simulink model "biasest_with_control"  (R2023b)
settings: Solver=FixedStepAuto  StartTime=0.0  StopTime=SIMTIME  FixedStep=SIMSTEP  RelTol=1e-3
values from neighbouring files (symbols this model uses):
  A = [z33,    eye(3) ... (first row only)    [bias_est.m]
  Aa = [A, Bv(:,1:3); zeros(3, 9)]    [bias_est.m]
  B = [z33, inv(M)]'    [bias_est.m]
  Ba = [B;zeros(3,3)]    [bias_est.m]
  beta_c = deg2rad(1)    [bias_est.m]
  bias = [1e4;1e3;0]    [bias_est.m]
  Bv = [z33 z33 ... (first row only)    [bias_est.m]
  C = [eye(3,6)]    [bias_est.m]
  Ca = [C, zeros(3,3)]    [bias_est.m]
  K2 = Kt2*Q    [bias_est.m]
  L = place(Aa', Ca', lambda_obs)'    [bias_est.m]
  ref = zeros(n_outputs, 1)    [bias_est.m]
  V_curr = 2    [bias_est.m]
  V_wind = 0    [bias_est.m]
  wave_ampl = [0, 0, 0]    [bias_est.m]
  wave_length = [70 70 70]    [bias_est.m]
  x0 = zeros(n_states,1)    [bias_est.m]
  xhat_0 = zeros(n_states+n_aug,1)    [bias_est.m]
undefined symbols (not defined in the file or in its folder): ocean_coeff, wind_coeff
settings Model: Creator=Lorenzo-Desk  LastModifiedBy=Lorenzo-Desk
settings DataIOCC: ReturnWorkspaceOutputs=off

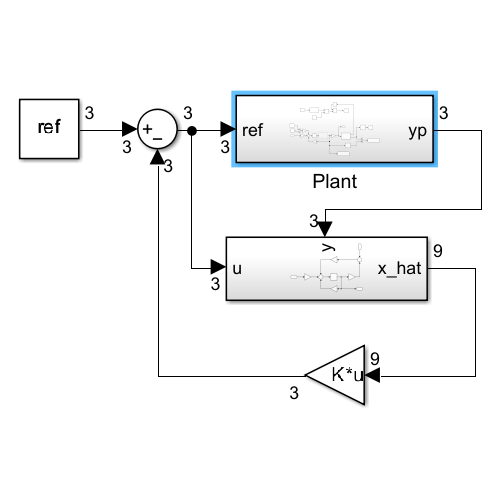
[thumbnail: Simulink's stored preview of the top-level diagram]
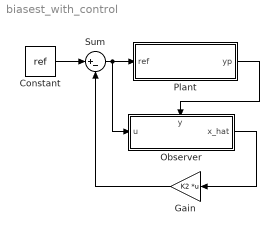
== system biasest_with_control ==
  Constant : Constant  Value=ref
  Gain : Gain  Gain=K2  Multiplication=Matrix(K*u)
  Observer : Subsystem
      settings: PortSchema="{\"entries\":[{\"content\":{\"sides\":[{\"content\":{\"connectorIds\":[\"In1\"]},\"type\":\"ConnectorPlacement.EquallySpacedRectSide\",\"uuid\":\"73eb13a4-821c-44f7-a0c5-8658f41102da\"},{\"content\":{\"connectorIds\":[\"Out1\"],\"side\":\"RIGHT\"},\"type\":\"ConnectorPlacement.EquallySpacedRectSide\",\"uuid\":\"46a10ada-d417-4d5f-8fe2-bf3b9a741608\"},{\"content\":{\"connectorIds\":[\"In2\"],\"side\":\"TOP\"},\"type\":\"ConnectorPlacement.EquallySpacedRectSide\",\"uuid\":\"761d0b5b-7137-4372-8030-4ca1ce843623\"}]},\"type\":\"ConnectorPlacement.EquallySpacedConnector\",\"uuid\":\"cfec28aa-9991-4d83-9aa1-5597ff8e72d9\"}],\"packageUris\":[\"http://schema.mathworks.com/mf0/Connector/R2020b\"],\"version\":\"1.0\"}"
  Plant : Subsystem
  Sum : Sum  Inputs=|+-
  wires:
  Plant/1(yp) -> Observer/2(y)
  Gain/1 -> Sum/2
  Observer/1(x_hat) -> Gain/1
  Constant/1 -> Sum/1
  Sum/1 -> Observer/1(u), Plant/1(ref)

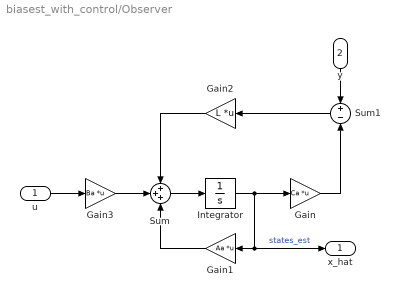
== system biasest_with_control/Observer ==
  u : Inport
  y : Inport  Port=2
  Gain : Gain  Gain=Ca  Multiplication=Matrix(K*u)
  Gain1 : Gain  Gain=Aa  Multiplication=Matrix(K*u)
  Gain2 : Gain  Gain=L  Multiplication=Matrix(K*u)
  Gain3 : Gain  Gain=Ba  Multiplication=Matrix(K*u)
  Integrator : Integrator  InitialCondition=xhat_0
  Sum : Sum  Inputs=+++
  Sum1 : Sum  Inputs=+|-
  x_hat : Outport
  wires:
  Integrator/1 -> Gain1/1, x_hat/1, Gain/1  "states_est"
  Sum/1 -> Integrator/1
  Gain/1 -> Sum1/2
  Sum1/1 -> Gain2/1
  Gain1/1 -> Sum/3
  Gain3/1 -> Sum/2
  u/1 -> Gain3/1
  y/1 -> Sum1/1
  Gain2/1 -> Sum/1

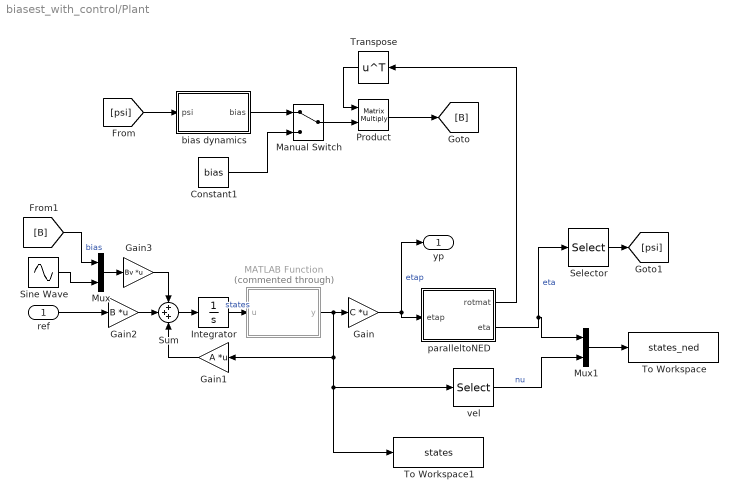
== system biasest_with_control/Plant ==
  ref : Inport
  Constant1 : Constant  Value=bias
  Gain : Gain  Gain=C  Multiplication=Matrix(K*u) (u vector)
  Gain1 : Gain  Gain=A  Multiplication=Matrix(K*u) (u vector)
  Gain2 : Gain  Gain=B  Multiplication=Matrix(K*u) (u vector)
  Gain3 : Gain  Gain=Bv  Multiplication=Matrix(K*u) (u vector)
  Integrator : Integrator  InitialCondition=x0
  MATLAB Function : MATLAB Function  Commented=through  TreatAsAtomicUnit=on
  Manual Switch : ManualSwitch
  Mux : Mux  Inputs=2
  Mux1 : Mux  Inputs=2
  Product : Product  Multiplication=Matrix(*)
  Selector : Selector  InputPortWidth=3  IndexOptions=Index vector (dialog)  Indices=[3]  OutputSizes=1
  Sine Wave : Sin  Amplitude=wave_ampl  Frequency=1./wave_length  SampleTime=0
  Sum : Sum  Inputs=+++
  To Workspace : ToWorkspace  VariableName=states_ned  SaveFormat=Timeseries  SampleTime=-1
  To Workspace1 : ToWorkspace  VariableName=states  SaveFormat=Timeseries  SampleTime=-1
  Transpose : Math  Operator=transpose
  bias dynamics : Subsystem
  paralleltoNED : MATLAB Function  TreatAsAtomicUnit=on
  vel : Selector  InputPortWidth=6  IndexOptions=Index vector (dialog)  Indices=[4 5 6]  OutputSizes=1
  yp : Outport
  wires:
  Transpose/1 -> Product/1
  vel/1 -> Mux1/2  "nu"
  Mux1/1 -> To Workspace/1
  paralleltoNED/1(rotmat) -> Transpose/1
  [psi] -> bias dynamics/1(psi)
  [B] -> Mux/1  "bias"
  Gain/1 -> paralleltoNED/1(etap), yp/1  "etap"
  Sine Wave/1 -> Mux/2
  Constant1/1 -> Manual Switch/2
  Mux/1 -> Gain3/1
  Integrator/1 -> MATLAB Function/1(u)  "states"
  ref/1 -> Gain2/1
  paralleltoNED/2(eta) -> Selector/1, Mux1/1  "eta"
  Gain1/1 -> Sum/3
  Sum/1 -> Integrator/1
  Gain2/1 -> Sum/2
  Selector/1 -> [psi]
  Gain3/1 -> Sum/1
  MATLAB Function/1(y) -> Gain/1, To Workspace1/1, vel/1, Gain1/1
  bias dynamics/1(bias) -> Manual Switch/1
  Manual Switch/1 -> Product/2
  Product/1 -> [B]

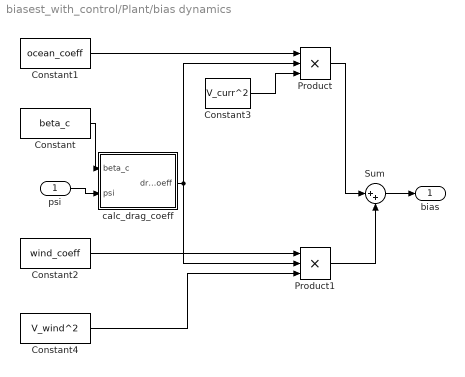
== system biasest_with_control/Plant/bias dynamics ==
  psi : Inport
  Constant : Constant  Value=beta_c
  Constant1 : Constant  Value=ocean_coeff
  Constant2 : Constant  Value=wind_coeff
  Constant3 : Constant  Value=V_curr^2
  Constant4 : Constant  Value=V_wind^2
  Product : Product  Inputs=3
  Product1 : Product  Inputs=3
  Sum : Sum  Inputs=|++
  calc_drag_coeff : MATLAB Function  TreatAsAtomicUnit=on
  bias : Outport
  wires:
  psi/1 -> calc_drag_coeff/2(psi)
  Constant/1 -> calc_drag_coeff/1(beta_c)
  Constant4/1 -> Product1/3
  Product/1 -> Sum/1
  Product1/1 -> Sum/2
  Sum/1 -> bias/1
  Constant1/1 -> Product/1
  calc_drag_coeff/1(drag_coeff) -> Product1/2, Product/2
  Constant3/1 -> Product/3
  Constant2/1 -> Product1/1

== matlab function biasest_with_control/Plant/paralleltoNED ==
  data: rotmat output; etap input; eta output
function [rotmat, eta] = fcn(etap)
    psip = etap(3);
    rotmat = [cos(psip), -sin(psip), 0; 
              sin(psip),  cos(psip), 0;
                      0,          0, 1];
    eta = rotmat*etap;
end

== matlab function biasest_with_control/Plant/MATLAB Function ==
  data: u input; y output
function y = fcn(u)
    u(3) = wrapTo2Pi(u(3)) - pi;
    y = u;
end

== matlab function biasest_with_control/Plant/bias dynamics/calc_drag_coeff ==
  data: beta_c input; drag_coeff output; psi input
function drag_coeff = fcn(beta_c, psi)
    angle_of_attack = psi-beta_c-pi;
    cx = 0.7;
    cy = 0.8; 
    cn = 0.15;
    Cx = -cx*cos(angle_of_attack);
    Cy = cy*sin(angle_of_attack);
    Cn = cn*sin(2*angle_of_attack);
    drag_coeff = [Cx, Cy, Cn]';
end
